simulink model "flujosok"  (Simulink 7.5)
settings: Solver=ode45  StartTime=0.0  StopTime=100  RelTol=1e-3
InitFcn:
  | 'para_inv_prechancado';
  | 'para_inv_prechancado';
  | 'volumen';
settings Model: Creator=vhandaluz  LastModifiedBy=Fer

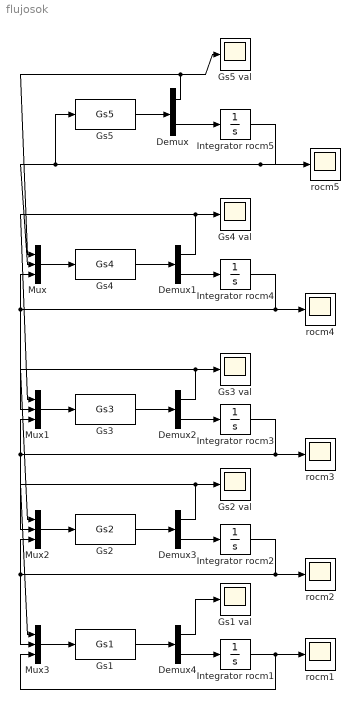
== system flujosok ==
  Demux{,1..4} (5 alike) : Demux  Outputs=2
  Gs1 : MATLABFcn  MATLABFcn=Gs1
  Gs1 val : Scope
      settings: SaveName=ScopeData8
  Gs2 : MATLABFcn  MATLABFcn=Gs2
  Gs2 val : Scope
      settings: SaveName=ScopeData6
  Gs3 : MATLABFcn  MATLABFcn=Gs3
  Gs3 val : Scope
      settings: SaveName=ScopeData4
  Gs4 : MATLABFcn  MATLABFcn=Gs4
  Gs4 val : Scope
      settings: SaveName=ScopeData2
  Gs5 : MATLABFcn  MATLABFcn=Gs5
  Gs5 val : Scope
  Integrator rocm{1..5} (5 alike) : Integrator  InitialCondition=1.6
  Mux{,1..3} (4 alike) : Mux  Inputs=3
  rocm{1..5} (5 alike) : Scope
      rocm1 settings: SaveName=ScopeData9
      rocm2 settings: SaveName=ScopeData7
      rocm3 settings: SaveName=ScopeData5
      rocm4 settings: SaveName=ScopeData3
  wires:
  Integrator rocm5/1 -> rocm5/1, Gs5/1, Mux/2
  Gs5/1 -> Demux/1
  Demux/2 -> Integrator rocm5/1
  Demux/1 -> Gs5 val/1, Mux/1
  Gs4/1 -> Demux1/1
  Demux1/2 -> Integrator rocm4/1
  Demux1/1 -> Gs4 val/1, Mux1/1
  Integrator rocm4/1 -> rocm4/1, Mux/3, Mux1/2
  Mux/1 -> Gs4/1
  Gs3/1 -> Demux2/1
  Demux2/2 -> Integrator rocm3/1
  Mux1/1 -> Gs3/1
  Demux2/1 -> Gs3 val/1, Mux2/1
  Integrator rocm3/1 -> rocm3/1, Mux1/3, Mux2/2
  Mux2/1 -> Gs2/1
  Gs2/1 -> Demux3/1
  Demux3/1 -> Gs2 val/1, Mux3/1
  Demux3/2 -> Integrator rocm2/1
  Integrator rocm2/1 -> rocm2/1, Mux2/3, Mux3/2
  Mux3/1 -> Gs1/1
  Gs1/1 -> Demux4/1
  Demux4/2 -> Integrator rocm1/1
  Demux4/1 -> Gs1 val/1
  Integrator rocm1/1 -> Mux3/3, rocm1/1
